simulink model "DC_motor_LQRp_c"  (R2015b)
settings: Solver=VariableStepAuto  StartTime=0.0  StopTime=10  MaxStep=1e-2  RelTol=1e-3
settings Model: Creator=mgreiff  LastModifiedBy=mgreiff
settings DebuggingCC: AlgebraicLoopMsg=none

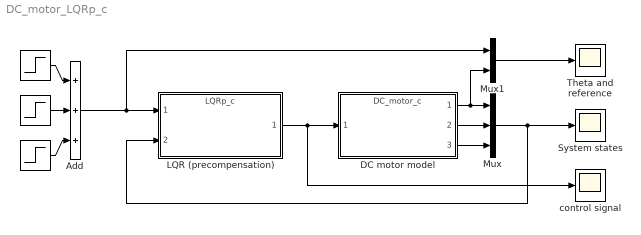
== system DC_motor_LQRp_c ==
  "  " : Step  Time=0  SampleTime=0
  "   " : Step  Time=4  After=-2  SampleTime=0
  "    " : Step  Time=8  SampleTime=0
  Add : Sum  Inputs=+++
  DC motor model : ModelReference  ModelNameDialog=DC_motor_c.slx  SimulationMode=Normal  ModelReferenceVersion=1.7  CopyOfModelName=DC_motor_c.slx
  LQR (precompensation) : ModelReference  ModelNameDialog=LQRp_c.slx  SimulationMode=Normal  ModelReferenceVersion=1.4  CopyOfModelName=LQRp_c.slx
  Mux : Mux  Inputs=3
  Mux1 : Mux  Inputs=2
  System states : Scope
  Theta and reference : Scope
  control signal : Scope
  wires:
  DC motor model/1 -> Mux1/2, Mux/1
  DC motor model/2 -> Mux/2
  DC motor model/3 -> Mux/3
  Mux/1 -> LQR (precompensation)/2, System states/1
  Add/1 -> LQR (precompensation)/1, Mux1/1
  Mux1/1 -> Theta and reference/1
  LQR (precompensation)/1 -> DC motor model/1, control signal/1
  "   "/1 -> Add/2
  "    "/1 -> Add/3
  "  "/1 -> Add/1
